simulink model "asynchronous_tau_2"  (R2022a)
settings: Solver=ode3  StartTime=0.0  StopTime=30  FixedStep=0.002  RelTol=1e-3  EnableMultiTasking=on
settings Model: Creator=Administrator  LastModifiedBy=11049
settings SolverCC: AlgebraicLoopSolver=TrustRegion
settings DataIOCC: LimitDataPoints=on  SaveFormat=Array  SignalLoggingSaveFormat=ModelDataLogs  ReturnWorkspaceOutputs=off
settings OptimizationCC: ExpressionDepthLimit=2147483647  LifeSpan=inf
settings DebuggingCC: UnderspecifiedInitializationDetection=Classic  MergeDetectMultiDrivingBlocksExec=none  FcnCallInpInsideContextMsg=warning  UnconnectedInputMsg=warning  UnconnectedOutputMsg=warning  UnconnectedLineMsg=warning  StateNameClashWarn=warning  SFUnexpectedBacktrackingDiag=warning  SFNoUnconditionalDefaultTransitionDiag=warning  SFExecutionAtInitializationDiag=none  SFMachineParentedDataDiag=warning  ArithmeticOperatorsInVariantConditions=warning
settings HardwareCC: ProdBitPerPointer=32  ProdBitPerSizeT=32  ProdBitPerPtrDiffT=32  ProdLargestAtomicFloat=None  ProdIntDivRoundTo=Undefined  ProdEndianess=Unspecified  ProdWordSize=32  ProdHWDeviceType=32-bit Generic
settings ModelReferenceCC: PropagateSignalLabelsOutOfModel=off
settings SFSimCC: SimUseLocalCustomCode=off  CustomCodeUndefinedFunction=UseInterfaceOnly
settings RTWCC: RTWUseLocalCustomCode=off
settings CodeAppCC: StateflowObjectComments=on
settings GRTTargetCC: TargetLangStandard=C89/C90 (ANSI)  CombineOutputUpdateFcns=off  GRTInterface=on
settings ConfigComp: CovMetricSettings=dw  CovSaveCumulativeToWorkspaceVar=on  CovSaveSingleToWorkspaceVar=on  CovExternalEMLEnable=off

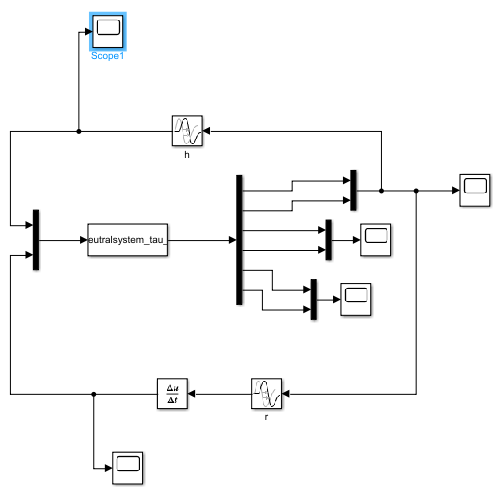
[thumbnail: Simulink's stored preview of the top-level diagram]
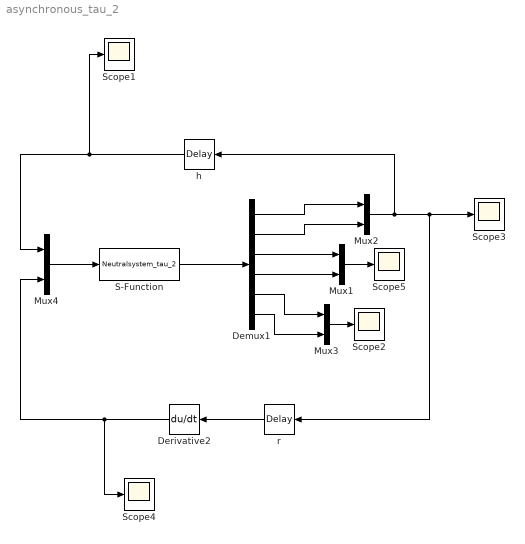
== system asynchronous_tau_2 ==
  Demux1 : Demux  Outputs=6
  Derivative2 : Derivative
  Mux{1..4} (4 alike) : Mux  Inputs=2
  S-Function : S-Function  FunctionName=Neutralsystem_tau_2  SFunctionDeploymentMode=off  EnableBusSupport=off
  Scope{1..5} (5 alike) : Scope
  h : TransportDelay  DelayTime=0.47878  BufferSize=4096
  r : TransportDelay  DelayTime=0.60665  BufferSize=999999
  wires:
  S-Function/1 -> Demux1/1
  Mux2/1 -> h/1, Scope3/1, r/1
  Mux4/1 -> S-Function/1
  Derivative2/1 -> Mux4/2, Scope4/1
  h/1 -> Mux4/1, Scope1/1
  r/1 -> Derivative2/1
  Demux1/1 -> Mux2/1
  Demux1/2 -> Mux2/2
  Demux1/3 -> Mux1/1
  Demux1/4 -> Mux1/2
  Mux1/1 -> Scope5/1
  Demux1/5 -> Mux3/1
  Demux1/6 -> Mux3/2
  Mux3/1 -> Scope2/1
